simulink model "dualConverter"  (R2024a)
settings: Solver=VariableStepAuto  StartTime=0.0  StopTime=5  FixedStep=0.01  RelTol=1e-3
libraries: spsThyristorLib x8, spsSeriesRLCBranchLib x2, spsACVoltageSourceLib x1, spsDCMachineLib x1, spsDCVoltageSourceLib x1, spsRMSLib x1, spsVoltageMeasurementLib x1, sps_lib x1
settings Model: Creator=farza  LastModifiedBy=farza

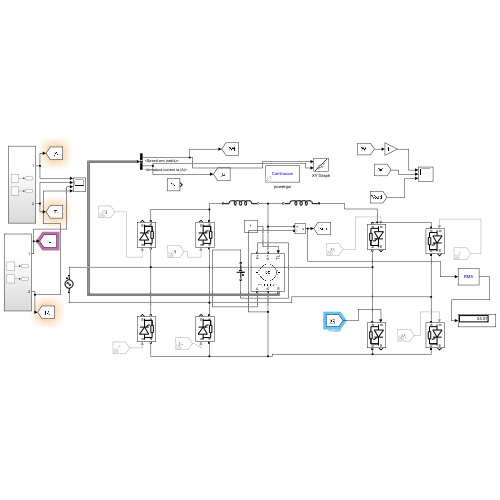
[thumbnail: Simulink's stored preview of the top-level diagram]
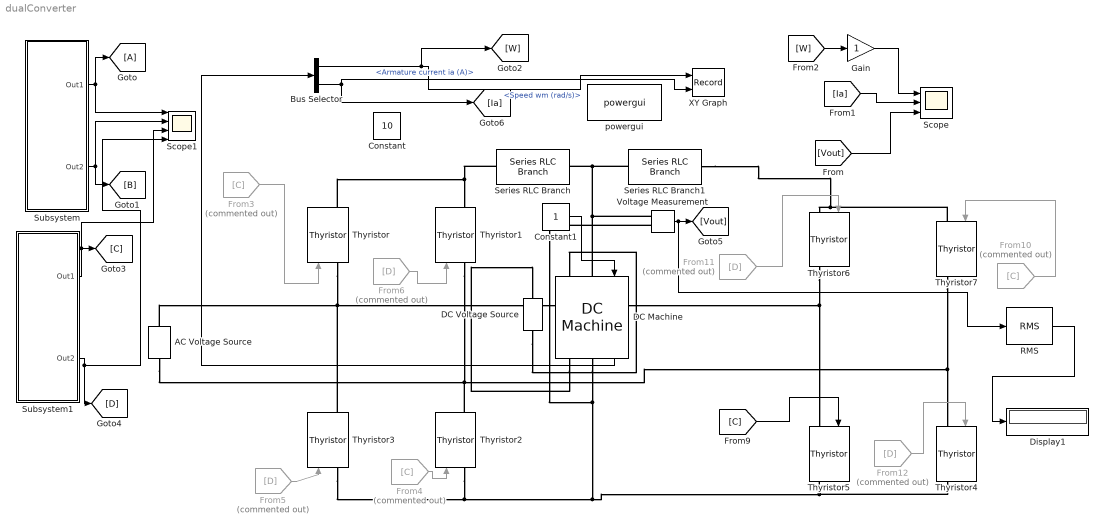
== system dualConverter ==
  AC Voltage Source : spsACVoltageSourceLib/AC Voltage Source  Amplitude=100  Phase=0  Frequency=50  SampleTime=0  Measurements=None  BusType=swing  Pref=10e3  Qref=0  Qmin=-inf  Qmax=+inf
  Bus Selector : BusSelector  OutputSignals=Speed wm (rad/s),Armature current ia (A)
  Constant : Constant  Value=10
  Constant1 : Constant
  DC Machine : spsDCMachineLib/DC Machine  PresetModel=No  MechanicalLoad=Torque TL  FieldType=Wound  ShowDetailedParameters=on  MeasurementBus=off  RLa="[ 0.6  0.012]"  RLf="[ 240  120]"  Laf=1.8  MachineConstant=Torque constant (N.m/A)  Ke=1.8  Kt=1.8  J=1  Bm=0  Tf=0  w0=1  Ifinit=0.416666666255433  TsPowergui=0  TsBlock=-1
  DC Voltage Source : spsDCVoltageSourceLib/DC Voltage Source  Amplitude=100  Measurements=None
  Display1 : Display
  From10 : From  Commented=on  GotoTag=C
  From{5..6,11..12} (4 alike) : From  Commented=on  GotoTag=D
  From3 : From  Commented=on  GotoTag=C
  From4 : From  Commented=on  GotoTag=C
  Gain : Gain
  Goto : Goto
  RMS : spsRMSLib/RMS  TrueRMS=on  Freq=60  RMSInit=120  Ts=0
  Scope : Scope  NumInputPorts=3
  Scope1 : Scope  NumInputPorts=4
  Series RLC Branch : spsSeriesRLCBranchLib/Series RLC Branch  LConnTagsString=__new0  RConnTagsString=__new0  BranchType=L  Resistance=1  Inductance=1e-3  SetiL0=off  InitialCurrent=0  Capacitance=1e-6  Setx0=off  InitialVoltage=0  Measurements=None
  Series RLC Branch1 : spsSeriesRLCBranchLib/Series RLC Branch  LConnTagsString=__new0  RConnTagsString=__new0  BranchType=L  Resistance=1  Inductance=1e-3  SetiL0=off  InitialCurrent=0  Capacitance=1e-6  Setx0=off  InitialVoltage=0  Measurements=None
  Subsystem : Subsystem
  Subsystem1 : Subsystem
  Thyristor{,1..7} (8 alike) : spsThyristorLib/Thyristor  Ron=0.001  Lon=0  Vf=0.8  IC=0  Rs=500  Cs=250e-9  Measurements=on
  Voltage Measurement : spsVoltageMeasurementLib/Voltage Measurement  PhasorSimulation=off  OutputType=Complex  PSBequivalent=0
  XY Graph : Record  FileSettingsInternal="{\"entries\":[{\"content\":{\"excelSettings\":{\"content\":{},\"type\":\"Streamout.ExcelSettings\"}},\"type\":\"Streamout.FileSettingStorage\",\"uuid\":\"\"}],\"packageUris\":[\"http:\\/\\/schema.mathworks.com\\/mf0\\/streamout_blocks\\/R2020a\"],\"version\":\"1.0\"}"  Layout=[1 1]  SignalsInternal="{\"entries\":[{\"content\":{\"signals\":[{\"content\":{\"blockPath\":[],\"dimensions\":[1],\"domain\":\"\",\"lineColor\":\"#ff6929\",\"lineWidth\":2,\"plots\":[ 1 ],\"port\":1,\"sid\":[\"\"],\"signalID\":1,\"signalName\":\"<Speed wm (rad\\/s)>\"},\"type\":\"RecordBlkView.Signal\",\"uuid\":\"\"},{\"content\":{\"blockPath\":[],\"dimensions\":[1],\"domain\":\"\",\"lineColor\":\"#b746ff\",\"lineWidth\":2,\"plots\":[ 1 ],\"port\":2,\"sid\":[\"\"],\"signalID\":2,\"signalName\":\"<Armature current ia (A)>\"},\"type\":\"RecordBlkView.Signal\",\"uuid\":\"\"}]},\"type\":\"RecordBlkView.InputSignals\",\"uuid\":\"\"}],\"packageUris\":[\"http:\\/\\/schema.mathworks.com\\/mf0\\/streamout_blocks\\/R2020a\"],\"version\":\"1.0\"}"  VisualizationBindings="{\"xyplotplugin\":{\"info\":[{\"series\":[{\"bindingParametersList\":[{\"parameter\":\"X-Axis\",\"signalID\":1,\"signalName\":\"<Speed wm (rad\\/s)>\"},{\"parameter\":\"Y-Axis\",\"signalID\":2,\"signalName\":\"<Armature current ia (A)>\"}],\"seriesID\":0}],\"subplotID\":1}]}}"  CompatibilityTag=XY
  powergui : sps_lib/powergui  Priority=1  SimulationMode=Continuous  SampleTime=50e-6  frequency=60  Iterations=50  frequencyindice=50  Pbase=100e6  ErrMax=1e-4  UnitsV=kV  UnitsW=MW  buscounter=0  FunctionMessages=off  echomessages=off  EnableUseOfTLC=off  CurrentSourceSwitches=off  DisableSnubberDevices=off  DisableRonSwitches=off  DisableVfSwitches=off  DisplayEquations=off  AutomaticDiscreteSolvers=off  SolverType=Tustin/Backward Euler (TBE)  Interpol=off  ExternalGateDelay=off  methode=off  Ts=100  x0status=blocks  SPID=on  SwTol=0  HookPort=off  NonlinearTolerance=1e-4  nMaxIteration=100  ContinueOnMaxIteration=off  RestoreLinks=warning  ResistiveCurrentMeasurement=off  Frange=[0:2:500]  Ylog=off  Xlog=on  ShowGrid=off  save=off  variable=ZData  structure=0  ZoomFFT=off  StartTime=0.0  cycles=1  DisplayStyle=1  fundamental=60  FreqAxis=off  MaxFrequency=1000  frequencyindicesteady=1  RmsSteady=1  display=off
  wires:
  Subsystem/1(Out1) -> Goto/1, Scope1/1
  Subsystem/2(Out2) -> [B], Scope1/2
  Subsystem1/1(Out1) -> Scope1/3, [C]
  Subsystem1/2(Out2) -> Scope1/4, [D]
  From3/1 -> Thyristor/1
  From4/1 -> Thyristor2/1
  From5/1 -> Thyristor3/1
  From6/1 -> Thyristor1/1
  From10/1 -> Thyristor7/1
  [C] -> Thyristor5/1
  From11/1 -> Thyristor6/1
  From12/1 -> Thyristor4/1
  Voltage Measurement/1 -> RMS/1, [Vout]
  Bus Selector/2 -> XY Graph/2, [Ia]  "<Armature current ia (A)>"
  [Vout] -> Scope/3
  DC Machine/1 -> Bus Selector/1
  Bus Selector/1 -> [W], XY Graph/1  "<Speed wm (rad/s)>"
  [Ia] -> Scope/2
  [W] -> Gain/1
  Gain/1 -> Scope/1
  Constant1/1 -> DC Machine/1
  RMS/1 -> Display1/1
  connections:
  Thyristor/RConn1 -- Thyristor1/RConn1 -- Series RLC Branch/LConn1
  Thyristor7/RConn1 -- Thyristor2/RConn1 -- Thyristor1/LConn1 -- AC Voltage Source/LConn1 -- Thyristor4/LConn1
  Thyristor7/LConn1 -- Series RLC Branch1/RConn1 -- Thyristor6/LConn1
  DC Voltage Source/RConn1 -- DC Machine/LConn2
  DC Machine/RConn2 -- DC Voltage Source/LConn1
  Series RLC Branch1/LConn1 -- Voltage Measurement/LConn1 -- DC Machine/LConn1 -- Series RLC Branch/RConn1
  Thyristor4/RConn1 -- Voltage Measurement/LConn2 -- DC Machine/RConn1 -- Thyristor2/LConn1 -- Thyristor3/LConn1 -- Thyristor5/RConn1
  Thyristor6/RConn1 -- Thyristor3/RConn1 -- Thyristor/LConn1 -- AC Voltage Source/RConn1 -- Thyristor5/LConn1

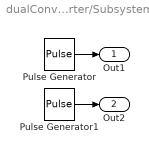
== system dualConverter/Subsystem ==
  Pulse Generator : DiscretePulseGenerator  PulseType=Time based  Amplitude=5  Period=1/50  PulseWidth=10  PhaseDelay=0.01/4
  Pulse Generator1 : DiscretePulseGenerator  PulseType=Time based  Amplitude=5  Period=1/50  PulseWidth=10  PhaseDelay=0.01+0.01/4
  Out1 : Outport
  Out2 : Outport  Port=2
  wires:
  Pulse Generator1/1 -> Out2/1
  Pulse Generator/1 -> Out1/1

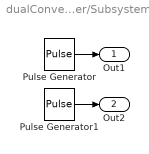
== system dualConverter/Subsystem1 ==
  Pulse Generator : DiscretePulseGenerator  PulseType=Time based  Amplitude=5  Period=1/50  PulseWidth=10  PhaseDelay=0.01-.01/4
  Pulse Generator1 : DiscretePulseGenerator  PulseType=Time based  Amplitude=5  Period=1/50  PulseWidth=10  PhaseDelay=0.01-.01/4+0.01
  Out1 : Outport
  Out2 : Outport  Port=2
  wires:
  Pulse Generator/1 -> Out1/1
  Pulse Generator1/1 -> Out2/1
